simulink model "example_controller_interface"  (R2016b)
settings: Solver=FixedStepDiscrete  StartTime=0.0  StopTime=inf  FixedStep=elmo_sample_time  RelTol=1e-3
values from neighbouring files (symbols this model uses):
  sample_time = 0.001    [daq_params_cmu.m]
undefined symbols (not defined in the file or in its folder): A_lpf_accelerometer, A_lpf_imu, B1_lpf_accelerometer, B1_lpf_imu, B2_lpf_accelerometer, B2_lpf_imu, g
libraries: simulink x2
settings Model: Creator=wmartin  LastModifiedBy=Will
settings SolverCC: EnableConcurrentExecution=on
settings DataIOCC: MaxDataPoints=1000000000  SaveFormat=StructureWithTime  SignalLogging=off  DSMLogging=off  VisualizeSimOutput=off
settings OptimizationCC: BlockReduction=off  OptimizeBlockIOStorage=off  BufferReuse=off  GlobalBufferReuse=off  ExpressionFolding=off  ExpressionDepthLimit=2147483647  LocalBlockOutputs=off  LifeSpan=inf  SimCompilerOptimization=on
settings DebuggingCC: UnderspecifiedInitializationDetection=Classic  MergeDetectMultiDrivingBlocksExec=none  SolverPrmCheckMsg=warning  StateNameClashWarn=warning  SFUnexpectedBacktrackingDiag=warning  SFNoUnconditionalDefaultTransitionDiag=warning  SFExecutionAtInitializationDiag=none
settings HardwareCC: ProdBitPerPointer=32  ProdBitPerSizeT=32  ProdBitPerPtrDiffT=32  ProdLargestAtomicFloat=None  ProdWordSize=32  ProdLongLongMode=on  ProdHWDeviceType=Generic->32-bit x86 compatible
settings ModelReferenceCC: UpdateModelReferenceTargets=IfOutOfDate  ModelReferenceNumInstancesAllowed=Single  ModelReferenceMinAlgLoopOccurrences=on  PropagateSignalLabelsOutOfModel=off
settings RTWCC: SystemTargetFile=slrt.tlc  TemplateMakefile=slrt_default_tmf  Description=Simulink Real-Time  RTWVerbose=off  RTWCompilerOptimization=on
settings CodeAppCC: MaxIdLength=256
settings SimulinkRealTimeCC: GeneratePreprocessorConditionals=Disable all  RL32LogBufSizeModifier=5e7
settings ConfigComp: CovMetricSettings=dw  CovHtmlReporting=on  CovSaveCumulativeToWorkspaceVar=on  CovSaveSingleToWorkspaceVar=on  CovExternalEMLEnable=off  CovSFcnEnable=off

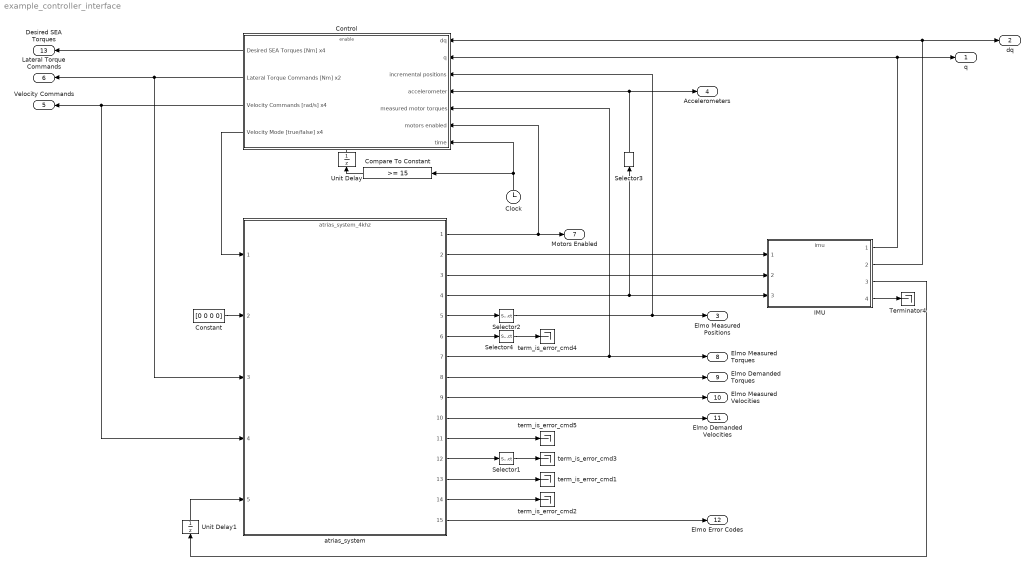
== system example_controller_interface ==
  Clock : Clock
  Compare To Constant : simulink/Logic and Bit Operations/Compare To Constant  relop=>=  const=15  OutDataTypeStr=boolean
  Constant : Constant  Value=[0 0 0 0]
  Control : Subsystem
  IMU : ModelReference  ModelNameDialog=imu  SimulationMode=Normal  ModelReferenceVersion=1.2458
  Selector1 : Selector  InputPortWidth=12  IndexOptions=Index vector (dialog)  Indices=[1 4 7 10]  OutputSizes=1
  Selector2 : Selector  InputPortWidth=6  IndexOptions=Index vector (dialog)  Indices=[1 2 3 4]  OutputSizes=1
  Selector3 : Selector  InputPortWidth=9  IndexOptions=Index vector (dialog)  Indices=[4 5 6]  OutputSizes=1
  Selector4 : Selector  InputPortWidth=6  IndexOptions=Index vector (dialog)  Indices=[1 2 3 4]  OutputSizes=1
  Terminator4 : Terminator
  Unit Delay : UnitDelay  SampleTime=-1
  Unit Delay1 : UnitDelay  SampleTime=-1
  atrias_system : ModelReference  ModelNameDialog=atrias_system_4khz  SimulationMode=Normal  ModelReferenceVersion=1.3099
  term_is_error_cmd{1..5} (5 alike) : Terminator
  q : Outport
  dq : Outport  Port=2
  Elmo Measured Positions : Outport  Port=3
  Accelerometers : Outport  Port=4
  Velocity Commands : Outport  Port=5
  Lateral Torque Commands : Outport  Port=6
  Motors Enabled : Outport  Port=7
  Elmo Measured Torques : Outport  Port=8
  Elmo Demanded Torques : Outport  Port=9
  Elmo Measured Velocities : Outport  Port=10
  Elmo Demanded Velocities : Outport  Port=11
  Elmo Error Codes : Outport  Port=12
  Desired SEA Torques : Outport  Port=13
  wires:
  Unit Delay/1 -> Control/Enable
  Compare To Constant/1 -> Unit Delay/1
  IMU/4 -> Terminator4/1
  IMU/3 -> Unit Delay1/1
  Selector3/1 -> Control/4(accelerometer), Accelerometers/1
  Unit Delay1/1 -> atrias_system/5
  Clock/1 -> Control/7(time), Compare To Constant/1
  atrias_system/2 -> IMU/1
  atrias_system/3 -> IMU/2
  atrias_system/5 -> Selector2/1
  atrias_system/6 -> Selector4/1
  atrias_system/7 -> Control/5(measured motor torques), Elmo Measured Torques/1
  atrias_system/8 -> Elmo Demanded Torques/1
  atrias_system/9 -> Elmo Measured Velocities/1
  atrias_system/10 -> Elmo Demanded Velocities/1
  atrias_system/11 -> term_is_error_cmd5/1
  atrias_system/12 -> Selector1/1
  atrias_system/13 -> term_is_error_cmd1/1
  atrias_system/14 -> term_is_error_cmd2/1
  Control/3(Velocity Commands [rad/s] x4) -> atrias_system/4, Velocity Commands/1
  atrias_system/1 -> Motors Enabled/1, Control/6(motors enabled)
  atrias_system/15 -> Elmo Error Codes/1
  Control/1(Desired SEA Torques [Nm] x4) -> Desired SEA Torques/1
  Control/2(Lateral Torque Commands [Nm] x2) -> atrias_system/3, Lateral Torque Commands/1
  Selector1/1 -> term_is_error_cmd3/1
  Selector4/1 -> term_is_error_cmd4/1
  IMU/1 -> q/1, Control/2(q)
  Selector2/1 -> Control/3(incremental positions), Elmo Measured Positions/1
  IMU/2 -> dq/1, Control/1(dq)
  atrias_system/4 -> IMU/3, Selector3/1
  Control/4(Velocity Mode [true/false] x4) -> atrias_system/1
  Constant/1 -> atrias_system/2

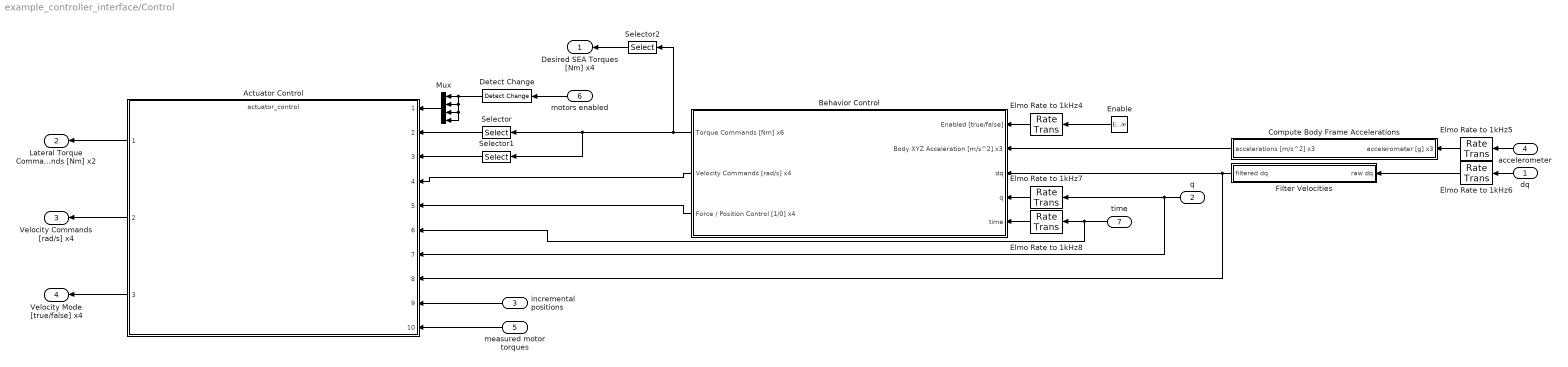
== system example_controller_interface/Control ==
  dq : Inport
  q : Inport  Port=2
  incremental positions : Inport  Port=3
  accelerometer : Inport  Port=4
  measured motor torques : Inport  Port=5
  motors enabled : Inport  Port=6
  time : Inport  Port=7
  Enable : EnablePort  StatesWhenEnabling=reset  PropagateVarSize=During execution  ShowOutputPort=on
  Actuator Control : ModelReference  ModelNameDialog=actuator_control  SimulationMode=Normal  ModelReferenceVersion=1.1457
  Behavior Control : Subsystem
  Compute Body Frame Accelerations : Subsystem
  Detect Change : simulink/Logic and Bit Operations/Detect Change  vinit=0  InputProcessing=Inherited  OutDataTypeStr=boolean
  Elmo Rate to 1kHz{4..8} (5 alike) : RateTransition  OutPortSampleTime=sample_time
  Filter Velocities : Subsystem
  Mux : Mux
  Selector : Selector  InputPortWidth=6  IndexOptions=Index vector (dialog)  Indices=[1 2 4 5]  OutputSizes=1
  Selector1 : Selector  InputPortWidth=6  IndexOptions=Index vector (dialog)  Indices=[3 6]  OutputSizes=1
  Selector2 : Selector  InputPortWidth=6  IndexOptions=Index vector (dialog)  Indices=[1 2 4 5]  OutputSizes=1
  Desired SEA Torques [Nm] x4 : Outport  InitialOutput=[0 0 0 0]
  Lateral Torque Commands [Nm] x2 : Outport  Port=2  InitialOutput=[0 0]
  Velocity Commands [rad/s] x4 : Outport  Port=3  InitialOutput=[0 0 0 0]
  Velocity Mode [true/false] x4 : Outport  Port=4  InitialOutput=[true true true true]
  wires:
  time/1 -> Actuator Control/6, Elmo Rate to 1kHz8/1
  Detect Change/1 -> Mux/1, Mux/2, Mux/3, Mux/4
  motors enabled/1 -> Detect Change/1
  Behavior Control/1(Torque Commands [Nm] x6) -> Selector2/1, Selector1/1, Selector/1
  Enable/1 -> Elmo Rate to 1kHz4/1
  Compute Body Frame Accelerations/1(accelerations [m/s^2] x3) -> Behavior Control/2(Body XYZ Acceleration [m/s^2] x3)
  accelerometer/1 -> Elmo Rate to 1kHz5/1
  Actuator Control/1 -> Lateral Torque Commands [Nm] x2/1
  q/1 -> Actuator Control/7, Elmo Rate to 1kHz7/1
  dq/1 -> Elmo Rate to 1kHz6/1
  Filter Velocities/1(filtered dq) -> Behavior Control/3(dq), Actuator Control/8
  incremental positions/1 -> Actuator Control/9
  measured motor torques/1 -> Actuator Control/10
  Selector/1 -> Actuator Control/2
  Behavior Control/2(Velocity Commands [rad/s] x4) -> Actuator Control/4
  Selector1/1 -> Actuator Control/3
  Mux/1 -> Actuator Control/1
  Elmo Rate to 1kHz5/1 -> Compute Body Frame Accelerations/1(accelerometer [g] x3)
  Elmo Rate to 1kHz6/1 -> Filter Velocities/1(raw dq)
  Elmo Rate to 1kHz7/1 -> Behavior Control/4(q)
  Elmo Rate to 1kHz8/1 -> Behavior Control/5(time)
  Behavior Control/3(Force / Position Control [1/0] x4) -> Actuator Control/5
  Elmo Rate to 1kHz4/1 -> Behavior Control/1(Enabled [true/false])
  Selector2/1 -> Desired SEA Torques [Nm] x4/1
  Actuator Control/3 -> Velocity Mode [true/false] x4/1
  Actuator Control/2 -> Velocity Commands [rad/s] x4/1

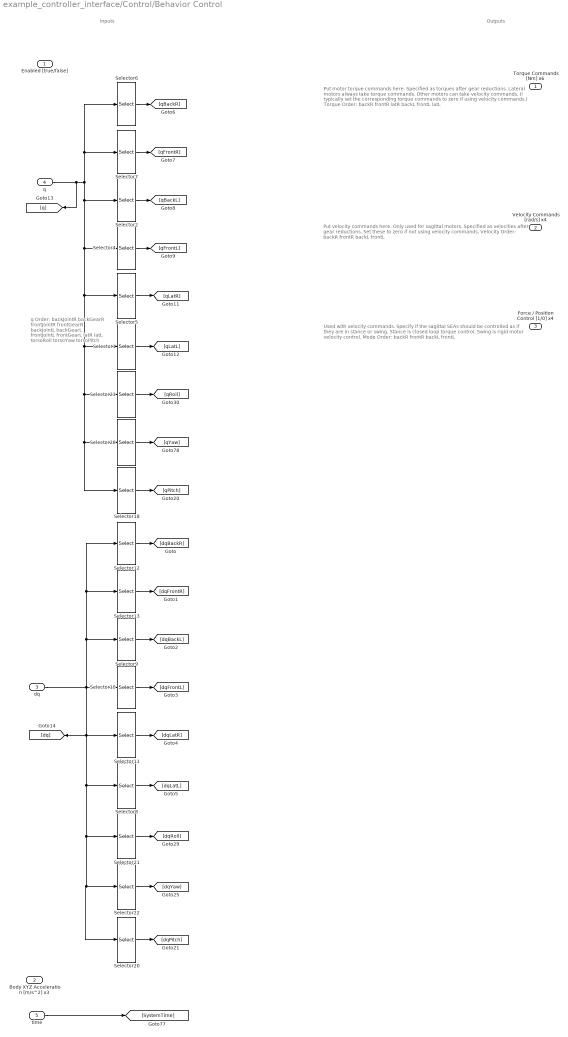
== system example_controller_interface/Control/Behavior Control ==
  note: Put motor torque commands here. Specified as torques after gear reductions. Lateral motors always take torque commands. Other motors can take velocity commands. (I typically set the corresponding torque commands to zero if using velocity commands.)
      |
      |
      | Torque Order:
      |
      | backR
      | frontR
      | latR
      | backL
      | frontL
      | latL
  note: q Order:
      |
      | backJointR
      | backGearR
      | frontJointR
      | frontGearR
      |
      | backJointL
      | backGearL
      | frontJointL
      | frontGearL
      |
      | latR
      | latL
      |
      | torsoRoll
      | torsoYaw
      | torsoPitch
  note: Inputs
  note: Outputs
  note: Put velocity commands here. Only used for sagittal motors. Specified as velocities after gear reductions. Set these to zero if not using velocity commands.
      |
      | Velocity Order:
      |
      | backR
      | frontR
      | backL
      | frontL
  note: Used with velocity commands. Specify if the sagittal SEAs should be controlled as if they are in stance or swing. Stance is closed loop torque control. Swing is rigid motor velocity control.
      |
      |
      | Mode Order:
      |
      | backR
      | frontR
      | backL
      | frontL
  Enabled [true/false] : Inport
  Body XYZ Acceleration [m/s^2] x3 : Inport  Port=2
  dq : Inport  Port=3
  q : Inport  Port=4
  time : Inport  Port=5
  Selector1 : Selector  InputPortWidth=13  IndexOptions=Index vector (dialog)  Indices=[10]  OutputSizes=1
  Selector10 : Selector  InputPortWidth=13  IndexOptions=Index vector (dialog)  Indices=[7 8]  OutputSizes=1
  Selector11 : Selector  InputPortWidth=13  IndexOptions=Index vector (dialog)  Indices=[9]  OutputSizes=1
  Selector12 : Selector  InputPortWidth=13  IndexOptions=Index vector (dialog)  Indices=[1 2]  OutputSizes=1
  Selector13 : Selector  InputPortWidth=13  IndexOptions=Index vector (dialog)  Indices=[3 4]  OutputSizes=1
  Selector18 : Selector  InputPortWidth=13  IndexOptions=Index vector (dialog)  Indices=[13]  OutputSizes=1
  Selector2 : Selector  InputPortWidth=13  IndexOptions=Index vector (dialog)  Indices=[5 6]  OutputSizes=1
  Selector20 : Selector  InputPortWidth=13  IndexOptions=Index vector (dialog)  Indices=[13]  OutputSizes=1
  Selector21 : Selector  InputPortWidth=13  IndexOptions=Index vector (dialog)  Indices=[11]  OutputSizes=1
  Selector22 : Selector  InputPortWidth=13  IndexOptions=Index vector (dialog)  Indices=[12]  OutputSizes=1
  Selector23 : Selector  InputPortWidth=13  IndexOptions=Index vector (dialog)  Indices=[11]  OutputSizes=1
  Selector28 : Selector  InputPortWidth=13  IndexOptions=Index vector (dialog)  Indices=[12]  OutputSizes=1
  Selector4 : Selector  InputPortWidth=13  IndexOptions=Index vector (dialog)  Indices=[7 8]  OutputSizes=1
  Selector5 : Selector  InputPortWidth=13  IndexOptions=Index vector (dialog)  Indices=[9]  OutputSizes=1
  Selector6 : Selector  InputPortWidth=13  IndexOptions=Index vector (dialog)  Indices=[1 2]  OutputSizes=1
  Selector7 : Selector  InputPortWidth=13  IndexOptions=Index vector (dialog)  Indices=[3 4]  OutputSizes=1
  Selector8 : Selector  InputPortWidth=13  IndexOptions=Index vector (dialog)  Indices=[10]  OutputSizes=1
  Selector9 : Selector  InputPortWidth=13  IndexOptions=Index vector (dialog)  Indices=[5 6]  OutputSizes=1
  Torque Commands [Nm] x6 : Outport  OutputWhenDisabled=reset  InitialOutput=[0 0 0 0 0 0]
  Velocity Commands [rad/s] x4 : Outport  Port=2  OutputWhenDisabled=reset  InitialOutput=[0 0 0 0 0 0]
  Force / Position Control [1/0] x4 : Outport  Port=3  OutputWhenDisabled=reset  InitialOutput=[0 0 0 0 0 0]
  wires:
  time/1 -> [SystemTime]
  dq/1 -> Selector9/1, Selector13/1, Selector12/1, Selector8/1, Selector22/1, Selector20/1, Selector21/1, Selector11/1, [dq], Selector10/1
  Selector21/1 -> [dqRoll]
  Selector22/1 -> [dqYaw]
  Selector20/1 -> [dqPitch]
  Selector10/1 -> [dqFrontL]
  Selector9/1 -> [dqBackL]
  Selector13/1 -> [dqFrontR]
  Selector12/1 -> [dqBackR]
  Selector11/1 -> [dqLatR]
  Selector8/1 -> [dqLatL]
  Selector28/1 -> [qYaw]
  Selector4/1 -> [qFrontL]
  Selector2/1 -> [qBackL]
  Selector7/1 -> [qFrontR]
  Selector6/1 -> [qBackR]
  Selector1/1 -> [qLatL]
  Selector5/1 -> [qLatR]
  q/1 -> Selector6/1, Selector7/1, Selector2/1, Selector4/1, Selector5/1, Selector18/1, Selector28/1, Selector23/1, Selector1/1, [q]
  Selector18/1 -> [qPitch]
  Selector23/1 -> [qRoll]

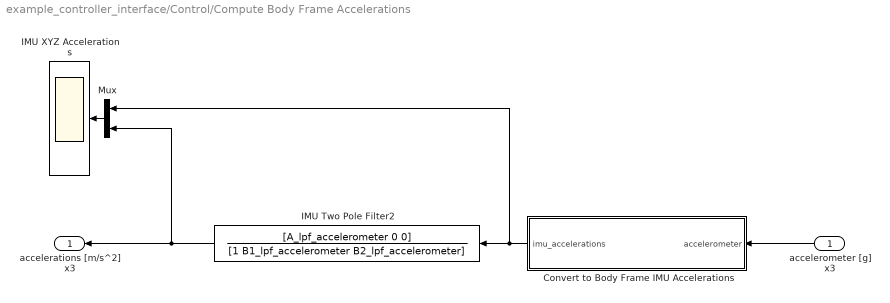
== system example_controller_interface/Control/Compute Body Frame Accelerations ==
  accelerometer [g] x3 : Inport
  Convert to Body Frame IMU Accelerations : MATLAB Function  TreatAsAtomicUnit=on
  IMU Two Pole Filter2 : DiscreteTransferFcn  Numerator=[A_lpf_accelerometer 0 0]  Denominator=[1 B1_lpf_accelerometer B2_lpf_accelerometer]  InitialStates=[0, 0, g; 0, 0, g]*15.277  SampleTime=sample_time
  IMU XYZ Accelerations : Scope
  Mux : Mux  Inputs=2
  accelerations [m/s^2] x3 : Outport
  wires:
  accelerometer [g] x3/1 -> Convert to Body Frame IMU Accelerations/1(accelerometer)
  Convert to Body Frame IMU Accelerations/1(imu_accelerations) -> Mux/1, IMU Two Pole Filter2/1
  Mux/1 -> IMU XYZ Accelerations/1
  IMU Two Pole Filter2/1 -> Mux/2, accelerations [m/s^2] x3/1

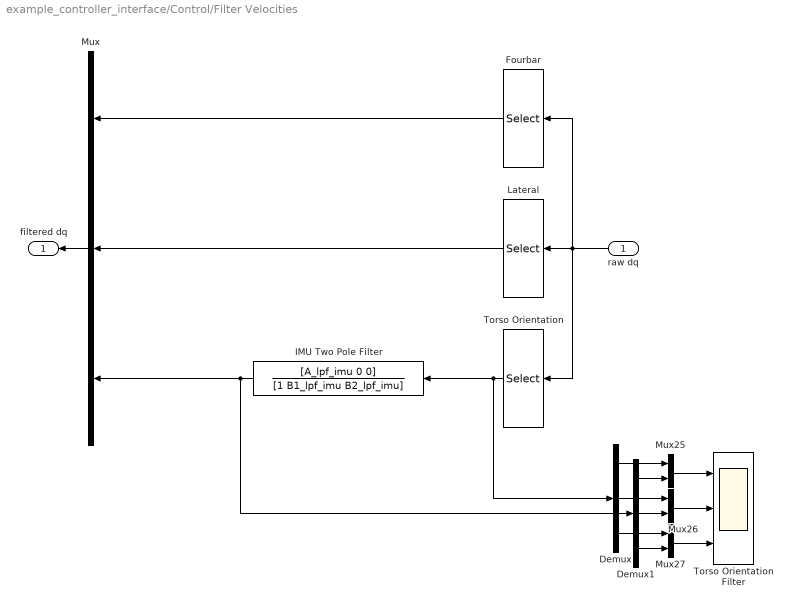
== system example_controller_interface/Control/Filter Velocities ==
  raw dq : Inport
  Demux : Demux  Outputs=3
  Demux1 : Demux  Outputs=3
  Fourbar : Selector  InputPortWidth=13  IndexOptions=Index vector (dialog)  Indices=[1 2 3 4 5 6 7 8]  OutputSizes=1
  IMU Two Pole Filter : DiscreteTransferFcn  Numerator=[A_lpf_imu 0 0]  Denominator=[1 B1_lpf_imu B2_lpf_imu]  SampleTime=sample_time
  Lateral : Selector  InputPortWidth=13  IndexOptions=Index vector (dialog)  Indices=[9 10]  OutputSizes=1
  Mux : Mux  Inputs=3
  Mux25 : Mux  Inputs=2
  Mux26 : Mux  Inputs=2
  Mux27 : Mux  Inputs=2
  Torso Orientation : Selector  InputPortWidth=13  IndexOptions=Index vector (dialog)  Indices=[11 12 13]  OutputSizes=1
  Torso Orientation Filter : Scope  NumInputPorts=3
  filtered dq : Outport
  wires:
  Demux1/3 -> Mux27/2
  Demux1/2 -> Mux26/2
  Demux1/1 -> Mux25/2
  Demux/3 -> Mux27/1
  Demux/2 -> Mux26/1
  Demux/1 -> Mux25/1
  Mux26/1 -> Torso Orientation Filter/2
  Mux27/1 -> Torso Orientation Filter/3
  Mux25/1 -> Torso Orientation Filter/1
  Lateral/1 -> Mux/2
  Torso Orientation/1 -> Demux/1, IMU Two Pole Filter/1
  raw dq/1 -> Lateral/1, Torso Orientation/1, Fourbar/1
  Mux/1 -> filtered dq/1
  IMU Two Pole Filter/1 -> Mux/3, Demux1/1
  Fourbar/1 -> Mux/1

== matlab function example_controller_interface/Control/Compute Body Frame Accelerations/Convert to Body Frame IMU Accelerations ==
  data: accelerometer input; imu_accelerations output; g parameter
function imu_accelerations = imu_to_body_frame(accelerometer, g)
    z_up_rotation = [1, 0, 0; 0, 0, 1; 0, -1, 0];
    align_xy_rotation = [sqrt(2)/2, -sqrt(2)/2, 0; sqrt(2)/2, sqrt(2)/2, 0; 0, 0, 1];
    imu_accelerations = g*z_up_rotation*align_xy_rotation*accelerometer;
end
